simulink model "Ques7Ex4_AkankshaMurali"  (R2023b)
settings: Solver=VariableStepAuto  StartTime=0.0  StopTime=10.0  RelTol=1e-3
settings Model: Creator=akank  LastModifiedBy=akank

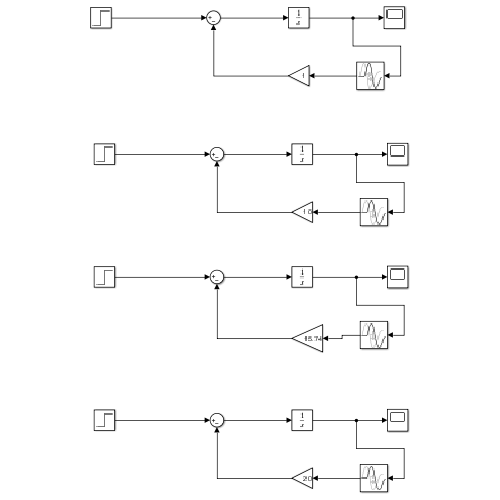
[thumbnail: Simulink's stored preview of the top-level diagram]
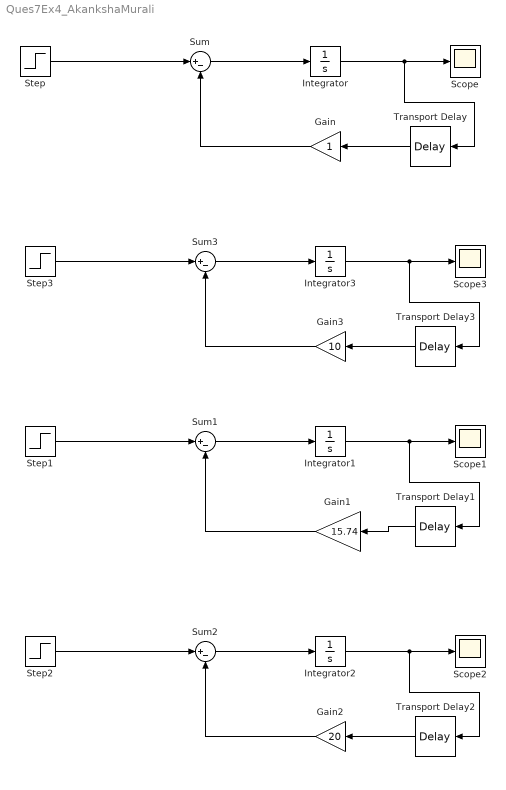
== system Ques7Ex4_AkankshaMurali ==
  Gain : Gain
  Gain1 : Gain  Gain=15.74
  Gain2 : Gain  Gain=20
  Gain3 : Gain  Gain=10
  Integrator{,1..3} (4 alike) : Integrator
  Scope{,1..3} (4 alike) : Scope
  Step{,1..3} (4 alike) : Step  Time=100  Before=0.001  After=0.001  SampleTime=0
  Sum{,1..3} (4 alike) : Sum  Inputs=|+-
  Transport Delay{,1..3} (4 alike) : TransportDelay  DelayTime=0.1
  wires:
  Sum1/1 -> Integrator1/1
  Step1/1 -> Sum1/1
  Transport Delay1/1 -> Gain1/1
  Integrator1/1 -> Transport Delay1/1, Scope1/1
  Gain1/1 -> Sum1/2
  Sum3/1 -> Integrator3/1
  Step3/1 -> Sum3/1
  Gain3/1 -> Sum3/2
  Sum/1 -> Integrator/1
  Integrator/1 -> Transport Delay/1, Scope/1
  Integrator3/1 -> Transport Delay3/1, Scope3/1
  Transport Delay3/1 -> Gain3/1
  Step/1 -> Sum/1
  Gain/1 -> Sum/2
  Transport Delay/1 -> Gain/1
  Transport Delay2/1 -> Gain2/1
  Gain2/1 -> Sum2/2
  Sum2/1 -> Integrator2/1
  Integrator2/1 -> Transport Delay2/1, Scope2/1
  Step2/1 -> Sum2/1
